simulink model "E1"  (R2023a)
settings: Solver=VariableStepAuto  StartTime=0.0  StopTime=0.08  MaxStep=1e-4  RelTol=1e-3
libraries: spsACVoltageSourceLib x2, spsMeanLib x2, spsSeriesRLCBranchLib x2, spsVoltageMeasurementLib x2, spsDetailedThyristorLib x1, spsDiodeLib x1, spspowerguiLib x1
settings Model: Creator=swara  LastModifiedBy=swara

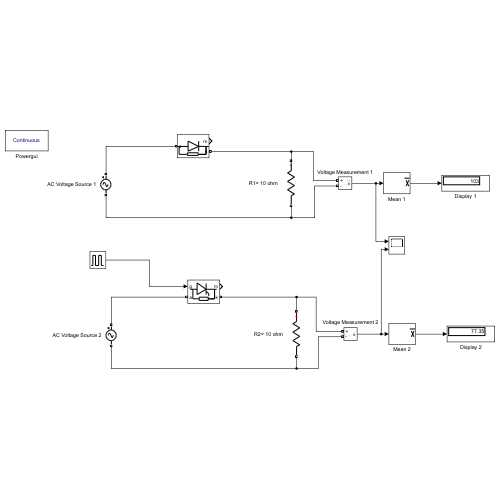
[thumbnail: Simulink's stored preview of the top-level diagram]
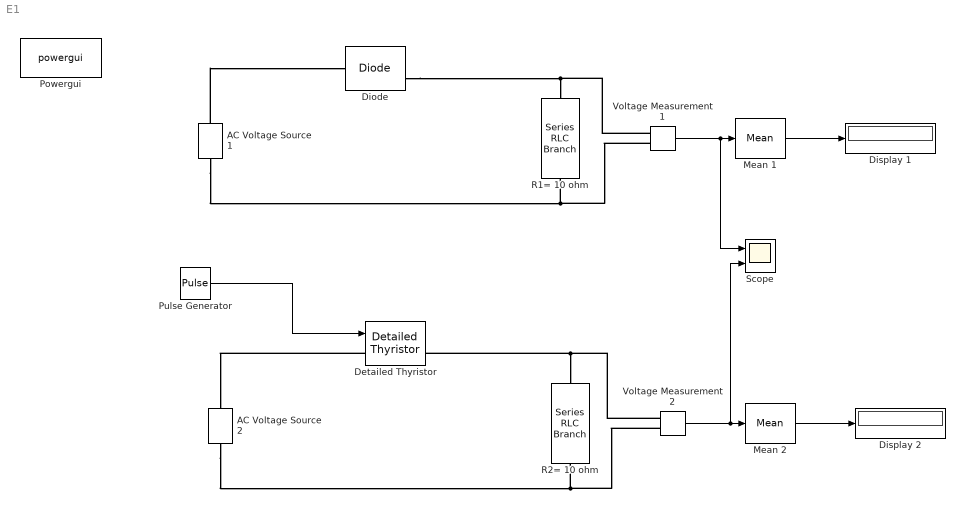
== system E1 ==
  AC Voltage Source 1 : spsACVoltageSourceLib/AC Voltage Source  Amplitude=325  Phase=0  Frequency=50  SampleTime=0  Measurements=None  BusType=swing  Pref=10e3  Qref=0  Qmin=-inf  Qmax=+inf
  AC Voltage Source 2 : spsACVoltageSourceLib/AC Voltage Source  Amplitude=325  Phase=0  Frequency=50  SampleTime=0  Measurements=None  BusType=swing  Pref=10e3  Qref=0  Qmin=-inf  Qmax=+inf
  Detailed Thyristor : spsDetailedThyristorLib/Detailed Thyristor  Ron=0.001  Lon=1e-3  Vf=0.8  IL=0.1  Tq=100e-6  IC=0  Rs=500  Cs=250e-9  Measurements=on
      settings: LibrarySourceBlock=sps_lib/Power Electronics/Detailed Thyristor
  Diode : spsDiodeLib/Diode  Ron=0.001  Lon=0  Vf=0.8  IC=0  UseSnubber=0  Rs=500  Cs=250e-9  Measurements=on
  Display 1 : Display
  Display 2 : Display
  Mean 1 : spsMeanLib/Mean  Freq=50  Vinit=0  Ts=0
  Mean 2 : spsMeanLib/Mean  Freq=50  Vinit=0  Ts=0
  Powergui : spspowerguiLib/powergui  Priority=1  SimulationMode=Continuous  SampleTime=50e-6  frequency=60  Iterations=50  frequencyindice=50  Pbase=100e6  ErrMax=1e-4  UnitsV=kV  UnitsW=MW  buscounter=0  FunctionMessages=off  echomessages=off  EnableUseOfTLC=off  CurrentSourceSwitches=off  DisableSnubberDevices=off  DisableRonSwitches=off  DisableVfSwitches=off  DisplayEquations=off  AutomaticDiscreteSolvers=off  SolverType=Tustin/Backward Euler (TBE)  Interpol=off  ExternalGateDelay=off  methode=off  Ts=100  x0status=blocks  SPID=on  SwTol=0  HookPort=off  NonlinearTolerance=1e-4  nMaxIteration=100  ContinueOnMaxIteration=off  RestoreLinks=warning  ResistiveCurrentMeasurement=off  Frange=[0:2:500]  Ylog=off  Xlog=on  ShowGrid=off  save=off  variable=ZData  structure=0  ZoomFFT=off  StartTime=0.0  cycles=1  DisplayStyle=1  fundamental=60  FreqAxis=off  MaxFrequency=1000  frequencyindicesteady=1  RmsSteady=1  display=off
  Pulse Generator : DiscretePulseGenerator  PulseType=Time based  Period=0.02  PulseWidth=5  PhaseDelay=60/360*0.02
  R1= 10 ohm : spsSeriesRLCBranchLib/Series RLC Branch  LConnTagsString=__new0  RConnTagsString=__new0  BranchType=R  Resistance=10  Inductance=1e-3  SetiL0=off  InitialCurrent=0  Capacitance=1e-6  Setx0=off  InitialVoltage=0  Measurements=None
  R2= 10 ohm : spsSeriesRLCBranchLib/Series RLC Branch  LConnTagsString=__new0  RConnTagsString=__new0  BranchType=R  Resistance=10  Inductance=1e-3  SetiL0=off  InitialCurrent=0  Capacitance=1e-6  Setx0=off  InitialVoltage=0  Measurements=None
  Scope : Scope  NumInputPorts=2
  Voltage Measurement 1 : spsVoltageMeasurementLib/Voltage Measurement  PhasorSimulation=off  OutputType=Complex  PSBequivalent=0
  Voltage Measurement 2 : spsVoltageMeasurementLib/Voltage Measurement  PhasorSimulation=off  OutputType=Complex  PSBequivalent=0
  wires:
  Voltage Measurement 1/1 -> Scope/1, Mean 1/1
  Mean 1/1 -> Display 1/1
  Mean 2/1 -> Display 2/1
  Voltage Measurement 2/1 -> Scope/2, Mean 2/1
  Pulse Generator/1 -> Detailed Thyristor/1
  connections:
  AC Voltage Source 1/RConn1 -- Diode/LConn1
  Diode/RConn1 -- Voltage Measurement 1/LConn1 -- R1= 10 ohm/LConn1
  AC Voltage Source 1/LConn1 -- Voltage Measurement 1/LConn2 -- R1= 10 ohm/RConn1
  Voltage Measurement 2/LConn1 -- R2= 10 ohm/LConn1 -- Detailed Thyristor/RConn1
  AC Voltage Source 2/LConn1 -- Voltage Measurement 2/LConn2 -- R2= 10 ohm/RConn1
  Detailed Thyristor/LConn1 -- AC Voltage Source 2/RConn1
